simulink model "heli_q8"  (R2020b)
settings: Solver=ode1  StartTime=0.0  StopTime=inf  FixedStep=0.002  RelTol=1e-3  EnableMultiTasking=on
PostLoadFcn:
  | qc_set_target_type(getConfigSet(bdroot, 'QUARC Default Target Configuration'));
values from neighbouring files (symbols this model uses):
  Cd = C_kalman    [init_heli_3_10.m]
  F = [K(1,1) K(1,3); K(2,1) K(2,3)]    [init_heli_3_10.m]    (also in init_heli_3_10_part2problem1.m)
  Joystick_gain_x = 1    [init_heli_3_10.m]    (also in init_heli_3_10_part2problem1.m)
  Joystick_gain_y = -1    [init_heli_3_10.m]    (also in init_heli_3_10_part2problem1.m)
  K = lqr(A,B,Q_lqr,R_lqr)    [init_heli_3_10.m]    (also in init_heli_3_10_part2problem1.m)
  P_0 = Qd    [init_heli_3_10.m]
  Qd = 0.000001*[1 0 0 0 0 0 ... (first row only)    [init_heli_3_10.m]
  Rd = [0.0067    0.0009    0.0073    0.0012    0.0013   -0.0002 ... (first row only)    [init_heli_3_10.m]
  v_s0 = 7.2    [init_heli_3_10.m]    (also in init_heli_3_10_part2problem1.m)
  x_0 = [0 ... (first row only)    [init_heli_3_10.m]
undefined symbols (not defined in the file or in its folder): Ad, Bd, HIL, qc_get_step_size
libraries: quarc_library x9
settings Model: SimulationMode=external  ExtModeTrigDuration=5000  Creator=Rchan  LastModifiedBy=danieana
settings SolverCC: PositivePriorityOrder=on
settings DataIOCC: LimitDataPoints=on  SaveFormat=Array  SignalLoggingSaveFormat=ModelDataLogs  ReturnWorkspaceOutputs=off
settings OptimizationCC: ExpressionDepthLimit=2147483647  InitFltsAndDblsToZero=on  LifeSpan=inf
settings DebuggingCC: SaveWithParameterizedLinksMsg=none  UnderspecifiedInitializationDetection=Classic  MergeDetectMultiDrivingBlocksExec=none  SolverPrmCheckMsg=warning  MultiTaskDSMMsg=warning  MultiTaskCondExecSysMsg=none  FcnCallInpInsideContextMsg=warning  AllowSymbolicDim=off  StateNameClashWarn=warning  SFUnexpectedBacktrackingDiag=warning  SFNoUnconditionalDefaultTransitionDiag=warning  SFExecutionAtInitializationDiag=none  ArithmeticOperatorsInVariantConditions=warning
settings HardwareCC: ProdBitPerPointer=32  ProdBitPerSizeT=32  ProdBitPerPtrDiffT=32  ProdLargestAtomicFloat=None  ProdIntDivRoundTo=Undefined  ProdEndianess=Unspecified  ProdWordSize=32  ProdHWDeviceType=32-bit Generic
settings ModelReferenceCC: PropagateSignalLabelsOutOfModel=off
settings SFSimCC: SimUseLocalCustomCode=off  CustomCodeUndefinedFunction=UseInterfaceOnly
settings RTWCC: Description=QUARC Win64 Target  SystemTargetFile=quarc_win64.tlc  TemplateMakefile=quarc_default_tmf  RTWUseLocalCustomCode=off
settings CodeAppCC: StateflowObjectComments=on
settings GRTTargetCC: TargetLangStandard=C89/C90 (ANSI)  ParMdlRefBuildCompliant=off  CompOptLevelCompliant=off  CombineOutputUpdateFcns=off  MatFileLogging=off  GRTInterface=on  UseToolchainInfoCompliant=off  ExtMode=on  ExtModeMexFile=quarc_comm
settings ConfigComp: CovMetricSettings=dw  CovSaveCumulativeToWorkspaceVar=on  CovSaveSingleToWorkspaceVar=on  CovExternalEMLEnable=off  CovSFcnEnable=off

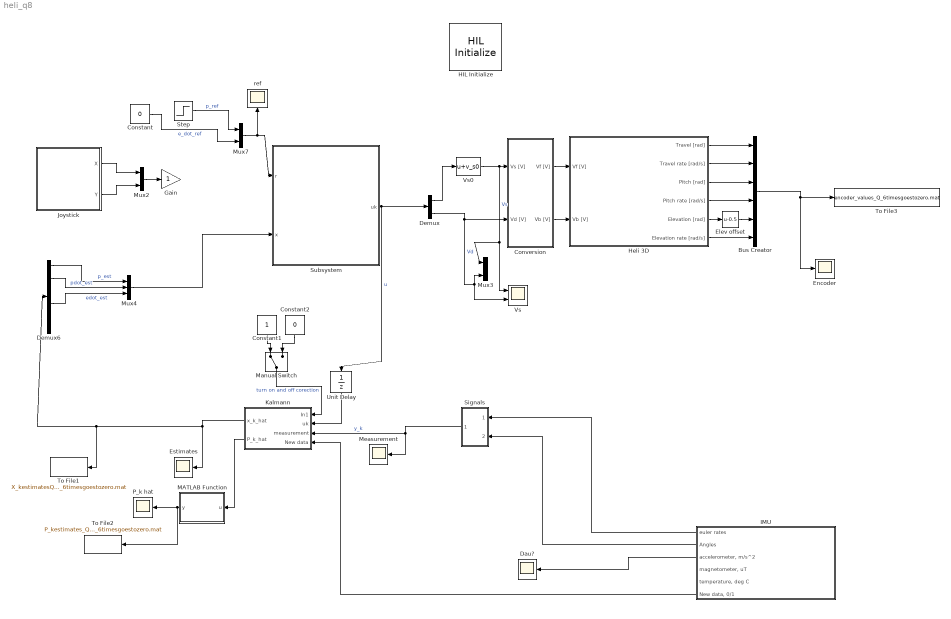
== system heli_q8 ==
  Bus Creator : BusCreator  Inputs=6
  Constant : Constant  Value=0
  Constant1 : Constant
  Constant2 : Constant  Value=0
  Conversion : Subsystem
  Dau? : Scope
  Demux : Demux  Outputs=2
  Demux6 : Demux  Outputs=6
  Elev offset : Bias  Bias=-0.5
  Encoder : Scope
  Estimates : Scope
  Gain : Gain
  HIL Initialize : quarc_library/Data Acquisition/Generic/Configuration/HIL Initialize  Priority=-99  object_name=HIL-1  board_type=q8_usb  board_number=0  board_options=update_rate=normal;decimation=1  exclusive=off  active=off  hardware_clocks=[0:2]  clock_modes=[]  initial_clock_frequencies=[]  set_clock_params_at_start=off  set_clock_params_at_switch_in=off  set_clock_frequencies_at_start=off  set_clock_frequencies_at_switch_in=off  analog_input_channels=[0:7]  analog_input_configurations=[]  analog_input_maximums=10  analog_input_minimums=-10  set_analog_input_params_at_start=on  set_analog_input_params_at_switch_in=off  analog_output_channels=[0:7]  analog_output_maximums=10  analog_output_minimums=-10  initial_analog_outputs=[0]  final_analog_outputs=[0]  watchdog_analog_outputs=0  set_analog_output_params_at_start=on  set_analog_output_params_at_switch_in=off  set_analog_outputs_at_start=on  set_analog_outputs_at_switch_in=off  set_analog_outputs_at_terminate=on  set_analog_outputs_at_switch_out=off  set_analog_outputs_on_watchdog=off  digital_input_channels=[]  digital_output_channels=[]  digital_output_configuration=[]  initial_digital_outputs=[1]  final_digital_outputs=[1]  watchdog_digital_outputs=[1]  set_digital_output_params_at_start=off  set_digital_output_params_at_switch_in=off  set_digital_outputs_at_start=on  set_digital_outputs_at_switch_in=off  set_digital_outputs_at_terminate=on  set_digital_outputs_at_switch_out=off  set_digital_outputs_on_watchdog=off  encoder_channels=[0:7]  quadrature=[4]  encoder_filter_frequency=[]  initial_encoder_counts=[0]  set_encoder_params_at_start=on  set_encoder_params_at_switch_in=off  set_encoder_counts_at_start=on  set_encoder_counts_at_switch_in=off  pwm_channels=[0:7]  pwm_modes=0  pwm_frequency=99.532799999999995e6/4095  pwm_configuration=[0]  pwm_alignment=[0]  pwm_polarity=[1]  pwm_leading_deadband=[0]  pwm_trailing_deadband=[0]  initial_pwm_outputs=[0]  final_pwm_outputs=[0]  watchdog_pwm_outputs=[0]  set_pwm_params_at_start=on  set_pwm_params_at_switch_in=off  set_pwm_outputs_at_start=on  set_pwm_outputs_at_switch_in=off  set_pwm_outputs_at_terminate=on  set_pwm_outputs_at_switch_out=off  set_pwm_outputs_on_watchdog=off  other_output_channels=[]  initial_other_outputs=[]  final_other_outputs=[]  watchdog_other_outputs=[]  set_other_outputs_at_start=off  set_other_outputs_at_switch_in=off  set_other_outputs_at_terminate=off  set_other_outputs_at_switch_out=off  set_other_outputs_on_watchdog=off
  Heli 3D : Subsystem
  IMU : Subsystem
  Joystick : Subsystem
  Kalmann : Subsystem
  MATLAB Function : MATLAB Function  TreatAsAtomicUnit=on
  Manual Switch : ManualSwitch
  Measurement : Scope
  Mux2 : Mux  Inputs=2
  Mux3 : Mux  Inputs=2
  Mux4 : Mux  Inputs=3
  Mux7 : Mux  Inputs=2
  P_k hat : Scope
  Signals : Subsystem
  Step : Step  Time=4  After=0.5  SampleTime=0
  Subsystem : Subsystem
  To File1 : ToFile  Filename=X_kestimatesQ_6timesgoestozero.mat
  To File2 : ToFile  Filename=P_kestimates_Q_6timesgoestozero.mat
  To File3 : ToFile  Filename=encoder_values_Q_6timesgoestozero.mat
  Unit Delay : UnitDelay  InitialCondition=[0;0]  SampleTime=-1  HasFrameUpgradeWarning=on
  Vs : Scope  NumInputPorts=2
  Vs0 : Bias  Bias=v_s0
  ref : Scope
  wires:
  Heli 3D/1(Travel [rad]) -> Bus Creator/1
  Heli 3D/2(Travel rate [rad/s]) -> Bus Creator/2
  Heli 3D/4(Pitch rate [rad/s]) -> Bus Creator/4
  Heli 3D/5(Elevation [rad]) -> Elev offset/1
  Heli 3D/6(Elevation rate [rad/s]) -> Bus Creator/6
  Elev offset/1 -> Bus Creator/5
  Vs0/1 -> Vs/1, Mux3/1, Conversion/1(Vs [V])  "Vs"
  Bus Creator/1 -> Encoder/1, To File3/1
  Demux/1 -> Vs0/1
  Heli 3D/3(Pitch [rad]) -> Bus Creator/3
  Subsystem/1(uk) -> Unit Delay/1, Demux/1  "u"
  Demux/2 -> Mux3/2, Vs/2, Conversion/2(Vd [V])  "Vd"
  Mux2/1 -> Gain/1
  Joystick/1(X) -> Mux2/1
  Joystick/2(Y) -> Mux2/2
  IMU/1(euler rates) -> Signals/1(In1)
  Demux6/1 -> Mux4/1  "p_est"
  Demux6/4 -> Mux4/3  "edot_est"
  Demux6/2 -> Mux4/2  "pdot_est"
  Mux4/1 -> Subsystem/2(x)
  Step/1 -> Mux7/1  "p_ref"
  Constant/1 -> Mux7/2  "e_dot_ref"
  Conversion/1(Vf [V]) -> Heli 3D/1(Vf [V])
  Conversion/2(Vb [V]) -> Heli 3D/2(Vb [V])
  IMU/6("New data, 0/1") -> Kalmann/4(New data)
  Kalmann/1(x_k_hat) -> Estimates/1, To File1/1, Demux6/1
  IMU/2(Angles) -> Signals/2(In2)
  Signals/1(Out1) -> Kalmann/3(measurement), Measurement/1  "y_k"
  IMU/3("accelerometer, m/s^2") -> Dau?/1
  Unit Delay/1 -> Kalmann/2(uk)
  Manual Switch/1 -> Kalmann/1(In1)  "turn on and off corection"
  Constant1/1 -> Manual Switch/1
  Constant2/1 -> Manual Switch/2
  Kalmann/2(P_k_hat) -> MATLAB Function/1(u)
  MATLAB Function/1(y) -> To File2/1, P_k hat/1
  Mux7/1 -> ref/1, Subsystem/1(r)

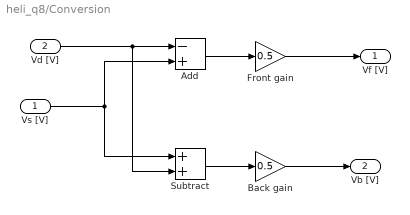
== system heli_q8/Conversion ==
  Vs [V] : Inport
  Vd [V] : Inport  Port=2
  Add : Sum  Inputs=-+
  Back gain : Gain  Gain=0.5
  Front gain : Gain  Gain=0.5
  Subtract : Sum
  Vf [V] : Outport
  Vb [V] : Outport  Port=2
  wires:
  Vd [V]/1 -> Subtract/2, Add/1
  Vs [V]/1 -> Subtract/1, Add/2
  Subtract/1 -> Back gain/1
  Back gain/1 -> Vb [V]/1
  Add/1 -> Front gain/1
  Front gain/1 -> Vf [V]/1

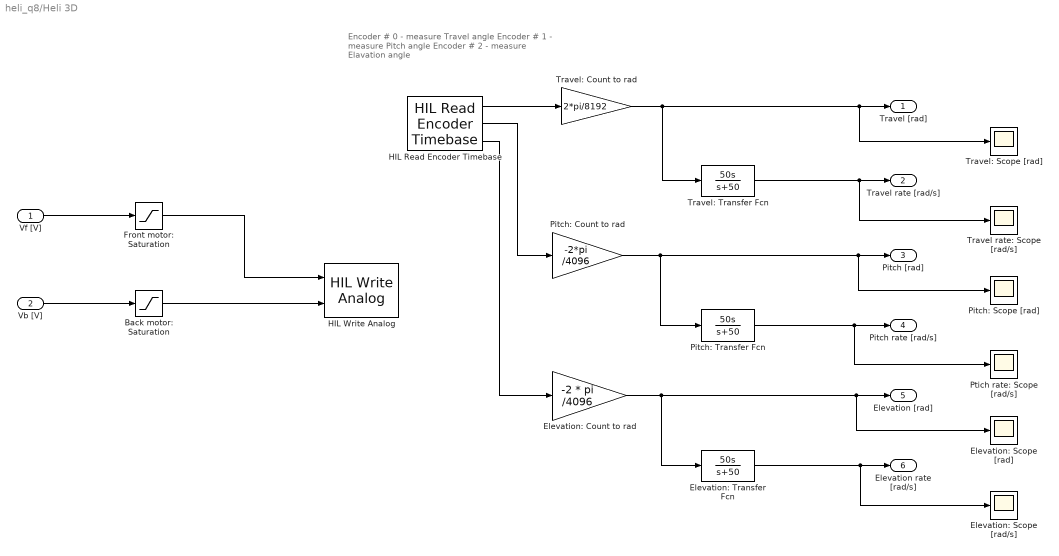
== system heli_q8/Heli 3D ==
  note: Encoder # 0 - measure Travel angle
      | Encoder # 1 - measure Pitch angle
      | Encoder # 2 - measure Elavation angle
  Vf [V] : Inport
  Vb [V] : Inport  Port=2
  Back motor: Saturation : Saturate  UpperLimit=5  LowerLimit=-5
  Elevation: Count to rad : Gain  Gain=-2 * pi /4096
  Elevation: Scope [rad/s] : Scope
  Elevation: Scope [rad] : Scope
  Elevation: Transfer Fcn : TransferFcn  Numerator=[50 0]  Denominator=[1 50]
  Front motor: Saturation : Saturate  UpperLimit=5  LowerLimit=-5
  HIL Read Encoder Timebase : quarc_library/Data Acquisition/Generic/Timebases/HIL Read Encoder Timebase  object_name=HIL-1  clock=0  channels=[0:2]  active=on  vector_output=off  data_type_mode=Inherit via back propagation  data_type=double  overflow_mode=Error on overflow  samples_in_buffer=max(ceil(1/qc_get_step_size), 1)
  HIL Write Analog : quarc_library/Data Acquisition/Generic/Immediate I//O/HIL Write Analog  object_name=HIL-1  channels=[0:1]  sample_time=-1  active=off  vector_input=off
  Pitch: Count to rad : Gain  Gain=-2*pi /4096
  Pitch: Scope [rad] : Scope
  Pitch: Transfer Fcn : TransferFcn  Numerator=[50 0]  Denominator=[1 50]
  Ptich rate: Scope [rad/s] : Scope
  Travel rate: Scope [rad/s] : Scope
  Travel: Count to rad : Gain  Gain=2*pi/8192
  Travel: Scope [rad] : Scope
  Travel: Transfer Fcn : TransferFcn  Numerator=[50 0]  Denominator=[1 50]
  Travel [rad] : Outport
  Travel rate [rad/s] : Outport  Port=2
  Pitch [rad] : Outport  Port=3
  Pitch rate [rad/s] : Outport  Port=4
  Elevation [rad] : Outport  Port=5
  Elevation rate [rad/s] : Outport  Port=6
  wires:
  HIL Read Encoder Timebase/1 -> Travel: Count to rad/1
  HIL Read Encoder Timebase/2 -> Pitch: Count to rad/1
  HIL Read Encoder Timebase/3 -> Elevation: Count to rad/1
  Travel: Count to rad/1 -> Travel: Scope [rad]/1, Travel [rad]/1, Travel: Transfer Fcn/1
  Travel: Transfer Fcn/1 -> Travel rate: Scope [rad/s]/1, Travel rate [rad/s]/1
  Pitch: Count to rad/1 -> Pitch: Transfer Fcn/1, Pitch: Scope [rad]/1, Pitch [rad]/1
  Pitch: Transfer Fcn/1 -> Ptich rate: Scope [rad/s]/1, Pitch rate [rad/s]/1
  Elevation: Count to rad/1 -> Elevation: Transfer Fcn/1, Elevation: Scope [rad]/1, Elevation [rad]/1
  Elevation: Transfer Fcn/1 -> Elevation: Scope [rad/s]/1, Elevation rate [rad/s]/1
  Vf [V]/1 -> Front motor: Saturation/1
  Vb [V]/1 -> Back motor: Saturation/1
  Front motor: Saturation/1 -> HIL Write Analog/1
  Back motor: Saturation/1 -> HIL Write Analog/2

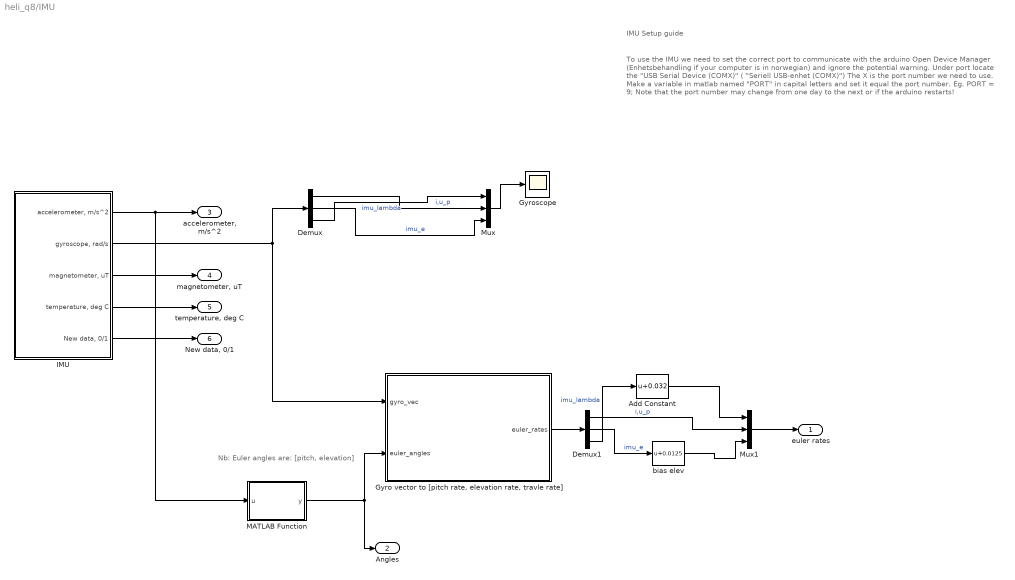
== system heli_q8/IMU ==
  note: Nb: Euler angles are: [pitch, elevation]
  note: IMU Setup guide
  note: To use the IMU we need to set the correct port to communicate with the arduino
      | Open Device Manager (Enhetsbehandling if your computer is in norwegian) and ignore the potential warning.
      | Under port locate the "USB Serial Device (COMX)" ( "Seriell USB-enhet (COMX)")
      | The X is the port number we need to use.
      |
      | Make a variable in matlab named "PORT" in capital letters and set it equal the port number.
      | Eg.
      | PORT = 9;
      |
      | Note that the port number may change from one day to the next or if the arduino restarts!
  Add Constant : Bias  Bias=0.032
  Demux : Demux  Outputs=3
  Demux1 : Demux  Outputs=3
  "Gyro vector to [pitch rate, elevation rate, travle rate]" : MATLAB Function  TreatAsAtomicUnit=on
  Gyroscope : Scope
  IMU : Subsystem
  MATLAB Function : MATLAB Function  TreatAsAtomicUnit=on
  Mux : Mux  Inputs=3
  Mux1 : Mux  Inputs=3
  bias elev : Bias  Bias=0.0125
  euler rates : Outport
  Angles : Outport  Port=2
  "accelerometer, m/s^2" : Outport  Port=3
  "magnetometer, uT" : Outport  Port=4
  "temperature, deg C" : Outport  Port=5
  "New data, 0/1" : Outport  Port=6
  wires:
  IMU/2("gyroscope, rad/s") -> Demux/1, "Gyro vector to [pitch rate, elevation rate, travle rate]"/1(gyro_vec)
  IMU/1("accelerometer, m/s^2") -> "accelerometer, m/s^2"/1, MATLAB Function/1(u)
  IMU/3("magnetometer, uT") -> "magnetometer, uT"/1
  IMU/4("temperature, deg C") -> "temperature, deg C"/1
  IMU/5("New data, 0/1") -> "New data, 0/1"/1
  Mux/1 -> Gyroscope/1
  Demux/2 -> Mux/3  "imu_e"
  Demux/3 -> Mux/1  "imu_lambda"
  Demux/1 -> Mux/2  "i,u_p"
  Demux1/2 -> bias elev/1  "imu_e"
  Mux1/1 -> euler rates/1
  Demux1/3 -> Add Constant/1  "imu_lambda"
  Demux1/1 -> Mux1/2  "i,u_p"
  "Gyro vector to [pitch rate, elevation rate, travle rate]"/1(euler_rates) -> Demux1/1
  Add Constant/1 -> Mux1/1
  bias elev/1 -> Mux1/3
  MATLAB Function/1(y) -> Angles/1, "Gyro vector to [pitch rate, elevation rate, travle rate]"/2(euler_angles)

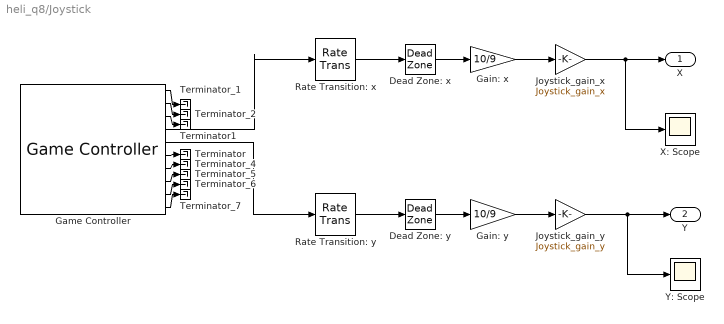
== system heli_q8/Joystick ==
  Dead Zone: x : DeadZone  LowerValue=-0.1  UpperValue=0.1  SaturateOnIntegerOverflow=on
  Dead Zone: y : DeadZone  LowerValue=-0.1  UpperValue=0.1  SaturateOnIntegerOverflow=on
  Gain: x : Gain  Gain=10/9
  Gain: y : Gain  Gain=10/9
  Game Controller : quarc_library/Devices/Peripherals/Target/Game Controller  controller=1  buffer_size=12  deadzone=[]  saturation=[]  sample_time=max(qc_get_step_size, 0.01)  auto_center=off  enabled=on
      settings: SourceProductName=QUARC Targets
  Joystick_gain_x : Gain  Gain=Joystick_gain_x
  Joystick_gain_y : Gain  Gain=Joystick_gain_y
  Rate Transition: x : RateTransition
  Rate Transition: y : RateTransition
  Terminator : Terminator
  Terminator1 : Terminator
  Terminator_{1..2,4..7} (6 alike) : Terminator
  X: Scope : Scope
  Y: Scope : Scope
  X : Outport
  Y : Outport  Port=2
  wires:
  Rate Transition: y/1 -> Dead Zone: y/1
  Rate Transition: x/1 -> Dead Zone: x/1
  Game Controller/5 -> Rate Transition: y/1
  Game Controller/4 -> Rate Transition: x/1
  Game Controller/1 -> Terminator_1/1
  Game Controller/2 -> Terminator_2/1
  Game Controller/7 -> Terminator_4/1
  Game Controller/8 -> Terminator_5/1
  Game Controller/9 -> Terminator_6/1
  Game Controller/10 -> Terminator_7/1
  Game Controller/3 -> Terminator1/1
  Game Controller/6 -> Terminator/1
  Dead Zone: x/1 -> Gain: x/1
  Dead Zone: y/1 -> Gain: y/1
  Gain: x/1 -> Joystick_gain_x/1
  Gain: y/1 -> Joystick_gain_y/1
  Joystick_gain_x/1 -> X/1, X: Scope/1
  Joystick_gain_y/1 -> Y: Scope/1, Y/1

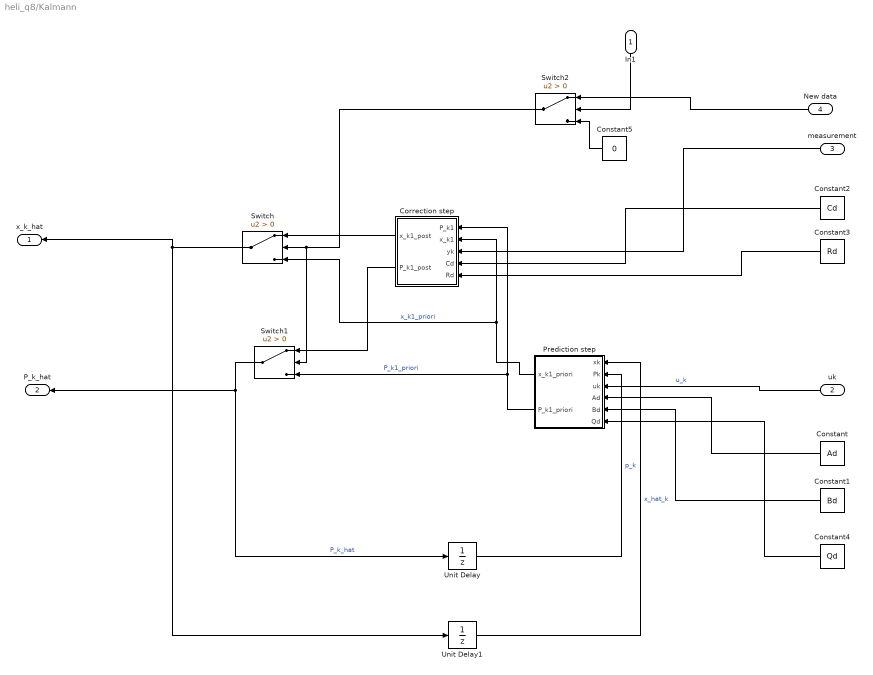
== system heli_q8/Kalmann ==
  In1 : Inport
  uk : Inport  Port=2
  measurement : Inport  Port=3
  New data : Inport  Port=4
  Constant : Constant  Value=Ad
  Constant1 : Constant  Value=Bd
  Constant2 : Constant  Value=Cd
  Constant3 : Constant  Value=Rd
  Constant4 : Constant  Value=Qd
  Constant5 : Constant  Value=0
  Correction step : MATLAB Function  TreatAsAtomicUnit=on
  Prediction step : MATLAB Function  TreatAsAtomicUnit=on
  Switch : Switch  Criteria=u2 > Threshold
  Switch1 : Switch  Criteria=u2 > Threshold
  Switch2 : Switch  Criteria=u2 > Threshold
  Unit Delay : UnitDelay  InitialCondition=P_0  SampleTime=-1  HasFrameUpgradeWarning=on
  Unit Delay1 : UnitDelay  InitialCondition=x_0  SampleTime=-1  HasFrameUpgradeWarning=on
  x_k_hat : Outport
  P_k_hat : Outport  Port=2
  wires:
  Unit Delay/1 -> Prediction step/2(Pk)  "p_k"
  Constant/1 -> Prediction step/4(Ad)
  Constant1/1 -> Prediction step/5(Bd)
  uk/1 -> Prediction step/3(uk)  "u_k"
  Prediction step/1(x_k1_priori) -> Switch/3, Correction step/2(x_k1)  "x_k1_priori"
  Prediction step/2(P_k1_priori) -> Correction step/1(P_k1), Switch1/3  "P_k1_priori"
  Constant2/1 -> Correction step/4(Cd)
  Constant3/1 -> Correction step/5(Rd)
  measurement/1 -> Correction step/3(yk)
  Correction step/1(x_k1_post) -> Switch/1
  Correction step/2(P_k1_post) -> Switch1/1
  Switch/1 -> x_k_hat/1, Unit Delay1/1
  Switch1/1 -> P_k_hat/1, Unit Delay/1  "P_k_hat"
  Constant4/1 -> Prediction step/6(Qd)
  Unit Delay1/1 -> Prediction step/1(xk)  "x_hat_k"
  New data/1 -> Switch2/1
  In1/1 -> Switch2/2
  Switch2/1 -> Switch1/2, Switch/2
  Constant5/1 -> Switch2/3

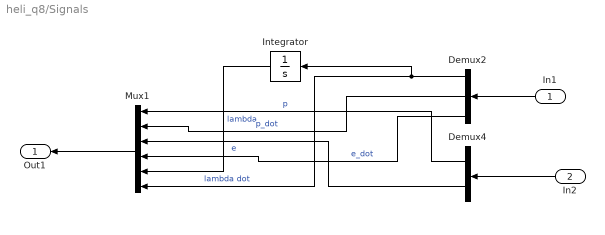
== system heli_q8/Signals ==
  In1 : Inport
  In2 : Inport  Port=2
  Demux2 : Demux  Outputs=3
  Demux4 : Demux  Outputs=2
  Integrator : Integrator
  Mux1 : Mux  Inputs=6
  Out1 : Outport
  wires:
  Mux1/1 -> Out1/1
  Demux2/1 -> Integrator/1, Mux1/6  "lambda dot"
  Integrator/1 -> Mux1/5  "lambda"
  Demux4/1 -> Mux1/1  "p"
  Demux2/2 -> Mux1/2  "p_dot"
  Demux4/2 -> Mux1/3  "e"
  Demux2/3 -> Mux1/4  "e_dot"
  In2/1 -> Demux4/1
  In1/1 -> Demux2/1

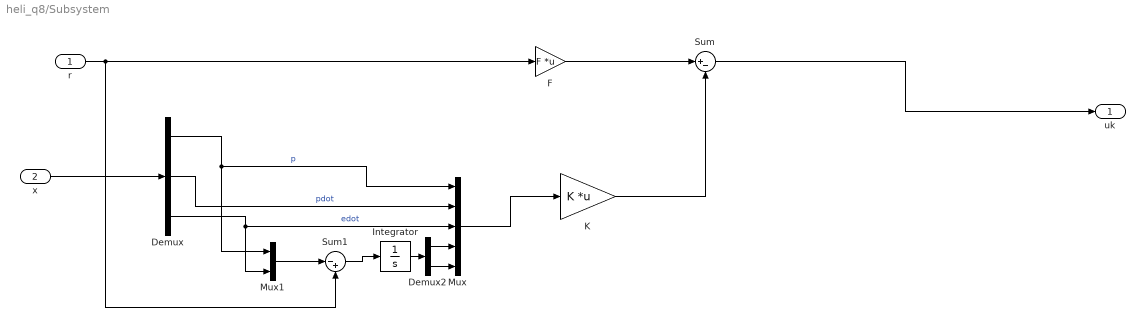
== system heli_q8/Subsystem ==
  r : Inport
  x : Inport  Port=2
  Demux : Demux  Outputs=3
  Demux2 : Demux  Outputs=2
  F : Gain  Gain=F  Multiplication=Matrix(K*u) (u vector)
  Integrator : Integrator
  K : Gain  Gain=K  Multiplication=Matrix(K*u) (u vector)
  Mux : Mux  Inputs=5
  Mux1 : Mux  Inputs=2
  Sum : Sum  Inputs=|+-
  Sum1 : Sum  Inputs=|-+
  uk : Outport
  wires:
  x/1 -> Demux/1
  Demux/2 -> Mux/2  "pdot"
  Demux/1 -> Mux/1, Mux1/1  "p"
  Demux/3 -> Mux1/2, Mux/3  "edot"
  Mux/1 -> K/1
  r/1 -> Sum1/2, F/1
  F/1 -> Sum/1
  K/1 -> Sum/2
  Sum/1 -> uk/1
  Mux1/1 -> Sum1/1
  Demux2/1 -> Mux/4
  Demux2/2 -> Mux/5
  Integrator/1 -> Demux2/1
  Sum1/1 -> Integrator/1

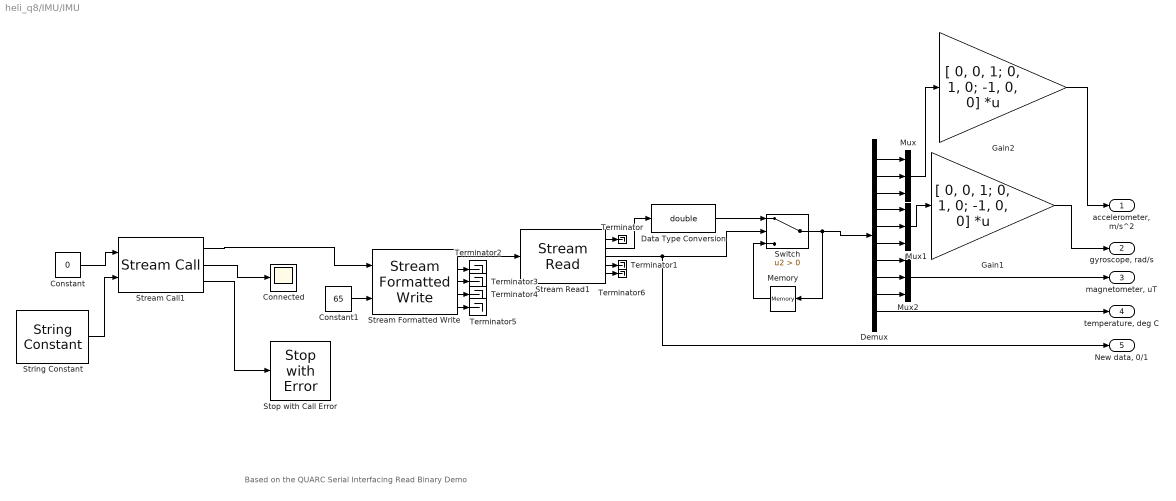
== system heli_q8/IMU/IMU ==
  note: Based on the QUARC Serial Interfacing Read Binary Demo
  Connected : Scope
  Constant : Constant  Value=0
  Constant1 : Constant  Value=65
  Data Type Conversion : DataTypeConversion  OutDataTypeStr=double
  Demux : Demux  Outputs=10
  Gain1 : Gain  Gain=[ 0, 0, 1; 0, 1, 0; -1, 0, 0]  Multiplication=Matrix(K*u) (u vector)
  Gain2 : Gain  Gain=[ 0, 0, 1; 0, 1, 0; -1, 0, 0]  Multiplication=Matrix(K*u) (u vector)
  Memory : Memory  InitialCondition=[0 0 0 0 0 0 0 0 0 0]
  Mux : Mux  Inputs=3
  Mux1 : Mux  Inputs=3
  Mux2 : Mux  Inputs=3
  Stop with Call Error : quarc_library/Sinks/Error Handling/Stop with Error  message_type=Interpret input as error code  message=Error occurred
      settings: SourceProductName=QUARC Targets
  Stream Call1 : quarc_library/Communications/Intermediate/Stream Call  uri_source=External input port  uri=serial://IMU:9?baud=115200,word=8,parity=none,stop=1,flow='none'  apply_uri_to_all_configs=on  send_buffer_size=8000  receive_buffer_size=8000  byte_order=little endian (Intel - LSB first)  sample_time=qc_get_step_size  non_blocking=on  active=off
      settings: SourceProductName=QUARC Targets
  Stream Formatted Write : quarc_library/Communications/Intermediate/Stream Formatted Write  format_string=%c\n  max_code_units=80  optimization=Minimizing latency
      settings: SourceProductName=QUARC Targets
  Stream Read1 : quarc_library/Communications/Intermediate/Stream Read  data_type=single  type_expr=BusObject  num_elements=10  receive_dims=off
      settings: SourceProductName=QUARC Targets
  String Constant : quarc_library/Strings/String Constant  string_value=qc_perform_substitutions('serial://IMU:%{PORT}?baud=115200,word=8,parity=none,stop=1')  evaluate_string=on  string_type=URI  max_length=255  sample_time=inf  variable_size=off
      settings: AttributesFormatString="\"serial://IMU:10?baud=115200,word=8,parity=none,stop=1\""  SourceProductName=QUARC Targets
  Switch : Switch  Criteria=u2 > Threshold
  Terminator{,1..6} (7 alike) : Terminator
  "accelerometer, m/s^2" : Outport
  "gyroscope, rad/s" : Outport  Port=2
  "magnetometer, uT" : Outport  Port=3
  "temperature, deg C" : Outport  Port=4
  "New data, 0/1" : Outport  Port=5
  wires:
  Switch/1 -> Memory/1, Demux/1
  Data Type Conversion/1 -> Switch/1
  Stream Read1/3 -> "New data, 0/1"/1, Switch/2
  Stream Formatted Write/1 -> Stream Read1/1
  Constant1/1 -> Stream Formatted Write/2
  Gain1/1 -> "gyroscope, rad/s"/1
  Gain2/1 -> "accelerometer, m/s^2"/1
  Stream Read1/4 -> Terminator1/1
  Demux/10 -> "temperature, deg C"/1
  Mux1/1 -> Gain1/1
  Stream Read1/2 -> Data Type Conversion/1
  Demux/7 -> Mux2/1
  Demux/8 -> Mux2/2
  Demux/9 -> Mux2/3
  Mux2/1 -> "magnetometer, uT"/1
  Demux/6 -> Mux1/3
  Demux/5 -> Mux1/2
  Demux/4 -> Mux1/1
  Mux/1 -> Gain2/1
  Demux/3 -> Mux/3
  Demux/1 -> Mux/1
  Demux/2 -> Mux/2
  Stream Read1/1 -> Terminator/1
  Stream Call1/1 -> Stream Formatted Write/1
  Constant/1 -> Stream Call1/1
  String Constant/1 -> Stream Call1/2
  Stream Call1/2 -> Connected/1
  Stream Call1/3 -> Stop with Call Error/1
  Memory/1 -> Switch/3
  Stream Formatted Write/2 -> Terminator2/1
  Stream Formatted Write/3 -> Terminator3/1
  Stream Formatted Write/4 -> Terminator4/1
  Stream Formatted Write/5 -> Terminator5/1
  Stream Read1/5 -> Terminator6/1

== matlab function heli_q8/IMU/MATLAB Function ==
  data: u input; y output
function y = ang_from_ax(u)
if u(3) == 0
    if u(2) < 0 
        p = pi/2;
    else
        p = -pi/2;
    end
else
    p = atan(u(2)/u(3));
end

den = sqrt(u(2)^2+u(3)^2);
if den == 0
    if u(1) < 0 
        e = pi/2;
    else
        e = -pi/2;
    end
else
    e = atan(u(1)/den);
end

y = [p; e];
end

== matlab function heli_q8/IMU/Gyro vector to [pitch rate, elevation rate, travle rate] ==
  data: gyro_vec input; euler_rates output; euler_angles input
function euler_rates = gyro_vec_to_euler_rates(gyro_vec,euler_angles)
%#codegen
    phi = euler_angles(1);
    theta = euler_angles(2);
    %psi = euler_angles(3);


    T = [1, sin(phi)*tan(theta), cos(phi)*tan(theta);
         0, cos(phi),            -sin(phi);
         0, sin(phi)/cos(theta), cos(phi)/cos(theta)]; 
euler_rates = T*gyro_vec;

== matlab function heli_q8/Kalmann/Prediction step ==
  data: xk input; x_k1_priori output; Pk input; uk input; Ad input; Bd input; P_k1_priori output; Qd input
function [x_k1_priori, P_k1_priori] = fcn(xk, Pk, uk, Ad, Bd,Qd)
x_k1_priori = xk;
P_k1_priori = Pk;


x_k1_priori = Ad*xk + Bd*uk;
P_k1_priori = Ad*Pk*Ad'+Qd;
end

== matlab function heli_q8/Kalmann/Correction step ==
  data: P_k1 input; x_k1_post output; x_k1 input; yk input; Cd input; Rd input; P_k1_post output
function [x_k1_post, P_k1_post] = fcn(P_k1, x_k1, yk, Cd, Rd)
% x_k1_post = x_k1;
% P_k1_post = P_k1;


L_k = (P_k1*Cd')/(Cd*P_k1*Cd'+Rd);
x_k1_post = x_k1+L_k*(yk-Cd*x_k1);
P_k1_post = (eye(6)-L_k*Cd)*P_k1*(eye(6)-L_k*Cd)'+L_k*Rd*L_k';
end

== matlab function heli_q8/MATLAB Function ==
  data: u input; y output
function y = fcn(u)
y = diag(u);
end
